simulink model "Micro_PMU_model"  (R2020b)
settings: Solver=VariableStepAuto  StartTime=0.0  StopTime=2  RelTol=1e-3  EnableMultiTasking=on
undefined symbols (not defined in the file): j, magnitude
libraries: powerlib_meascontrol x15, dsparch4 x3, dspsigops x3, powerlib x1
(part 1 of 3)
settings Model: Creator=Ahmed A.Elaziz  LastModifiedBy=Electronica Care
settings DataIOCC: ReturnWorkspaceOutputs=off
settings OptimizationCC: LifeSpan=inf
settings DebuggingCC: SFUnexpectedBacktrackingDiag=warning  SFNoUnconditionalDefaultTransitionDiag=warning  ArithmeticOperatorsInVariantConditions=warning
settings SFSimCC: SimUseLocalCustomCode=off  CustomCodeUndefinedFunction=UseInterfaceOnly
settings RTWCC: RTWUseLocalCustomCode=off
settings CodeAppCC: StateflowObjectComments=on
settings GRTTargetCC: TargetLangStandard=C89/C90 (ANSI)
settings ConfigComp: CovMetricSettings=dw  CovSaveCumulativeToWorkspaceVar=on  CovSaveSingleToWorkspaceVar=on  CovExternalEMLEnable=off

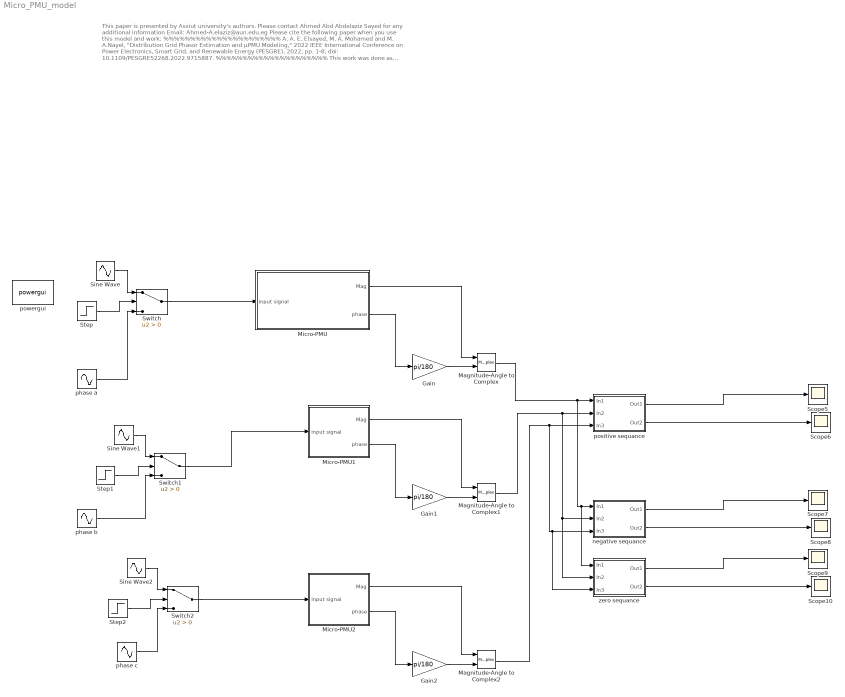
== system Micro_PMU_model ==
  note: This paper is presented by Assiut university's authors.
      | Please contact Ahmed Abd Abdelaziz Sayed for any additional information
      | Email: Ahmed-A.elaziz@aun.edu.eg
      |
      | Please cite the following paper when you use this model and work:
      | %%%%%%%%%%%%%%%%%%%%%%
      | A. A. E. Elsayed, M. A. Mohamed and M. A.Nayel,
      | "Distribution Grid Phasor Estimation and μPMU Modeling,"
      | 2022 IEEE International Conference on Power Electronics, Smart Grid, and Renewable Energy (PESGRE),
      | 2022, pp. 1-8, doi: 10.1109/PESGRE52268.2022.9715887.
      | %%%%%%%%%%%%%%%%%%%%%
      | This work was done as part of the research project “
      | Smart Monitoring system for Distribution Power Grid ”
      | supported by the Egyptian National Telecom Regulatory
      | Authority (NTRA).
      |
      | I hope this model and material are useful for you!!
      | Best wishes.
  Gain : Gain  Gain=pi/180
  Gain1 : Gain  Gain=pi/180
  Gain2 : Gain  Gain=pi/180
  Magnitude-Angle to Complex : MagnitudeAngleToComplex
  Magnitude-Angle to Complex1 : MagnitudeAngleToComplex
  Magnitude-Angle to Complex2 : MagnitudeAngleToComplex
  Micro-PMU : Subsystem
      mask Display: image('C:\Users\Ahmed A.Elaziz\Desktop\microPMU.png');
  Micro-PMU1 : Subsystem
      mask Display: image('C:\Users\Ahmed A.Elaziz\Desktop\microPMU.png');
  Micro-PMU2 : Subsystem
      mask Display: image('C:\Users\Ahmed A.Elaziz\Desktop\microPMU.png');
  Scope{5..10} (6 alike) : Scope
  Sine Wave : Sin  Frequency=2*pi*60  Phase=0/180*pi  SampleTime=0
  Sine Wave1 : Sin  Frequency=2*pi*60  Phase=-120/180*pi  SampleTime=0
  Sine Wave2 : Sin  Frequency=2*pi*60  Phase=120/180*pi  SampleTime=0
  Step : Step  Before=1  After=0  SampleTime=0
  Step1 : Step  Before=1  After=0  SampleTime=0
  Step2 : Step  Before=1  After=0  SampleTime=0
  Switch : Switch  Criteria=u2 > Threshold
  Switch1 : Switch  Criteria=u2 > Threshold
  Switch2 : Switch  Criteria=u2 > Threshold
  negative sequance : Subsystem
  phase a : Sin  Frequency=2*pi*59  Phase=0/180*pi  SampleTime=0
  phase b : Sin  Frequency=2*pi*59  Phase=-120/180*pi  SampleTime=0
  phase c : Sin  Frequency=2*pi*59  Phase=120/180*pi  SampleTime=0
  "positive sequance " : Subsystem
  powergui : powerlib/powergui  Priority=1  SimulationMode=Continuous  SampleTime=50e-6  frequency=60  Iterations=50  frequencyindice=60  Pbase=100e6  ErrMax=1e-4  UnitsV=kV  UnitsW=MW  buscounter=0  FunctionMessages=off  echomessages=off  EnableUseOfTLC=off  CurrentSourceSwitches=off  DisableSnubberDevices=off  DisableRonSwitches=off  DisableVfSwitches=off  DisplayEquations=off  AutomaticDiscreteSolvers=off  SolverType=Tustin/Backward Euler (TBE)  Interpol=off  ExternalGateDelay=off  methode=off  Ts=10  x0status=blocks  SPID=off  SwTol=0  HookPort=off  NonlinearTolerance=1e-4  nMaxIteration=100  ContinueOnMaxIteration=off  RestoreLinks=warning  ResistiveCurrentMeasurement=off  Frange=[0:2:500]  Ylog=off  Xlog=on  ShowGrid=off  save=off  variable=ZData  structure=0  ZoomFFT=off  StartTime=0.0  cycles=1  DisplayStyle=1  fundamental=60  FreqAxis=off  MaxFrequency=1000  frequencyindicesteady=1  RmsSteady=1  display=off
  "zero sequance " : Subsystem
  wires:
  Sine Wave1/1 -> Switch1/1
  "positive sequance "/1(Out1) -> Scope5/1
  Micro-PMU1/2(phase) -> Gain1/1
  Step/1 -> Switch/2
  Micro-PMU1/1(Mag) -> Magnitude-Angle to Complex1/1
  Micro-PMU/2(phase) -> Gain/1
  Sine Wave/1 -> Switch/1
  Gain2/1 -> Magnitude-Angle to Complex2/2
  Micro-PMU/1(Mag) -> Magnitude-Angle to Complex/1
  Gain1/1 -> Magnitude-Angle to Complex1/2
  negative sequance/1(Out1) -> Scope7/1
  Magnitude-Angle to Complex1/1 -> "zero sequance "/2(In2), negative sequance/2(In2), "positive sequance "/2(In2)
  Magnitude-Angle to Complex2/1 -> "zero sequance "/3(In3), negative sequance/3(In3), "positive sequance "/3(In3)
  "positive sequance "/2(Out2) -> Scope6/1
  Magnitude-Angle to Complex/1 -> "zero sequance "/1(In1), negative sequance/1(In1), "positive sequance "/1(In1)
  "zero sequance "/1(Out1) -> Scope9/1
  Step2/1 -> Switch2/2
  "zero sequance "/2(Out2) -> Scope10/1
  negative sequance/2(Out2) -> Scope8/1
  phase c/1 -> Switch2/3
  Step1/1 -> Switch1/2
  Switch2/1 -> Micro-PMU2/1(input signal)
  Sine Wave2/1 -> Switch2/1
  phase a/1 -> Switch/3
  Switch1/1 -> Micro-PMU1/1(input signal)
  Micro-PMU2/2(phase) -> Gain2/1
  Switch/1 -> Micro-PMU/1(input signal)
  phase b/1 -> Switch1/3
  Gain/1 -> Magnitude-Angle to Complex/2
  Micro-PMU2/1(Mag) -> Magnitude-Angle to Complex2/1

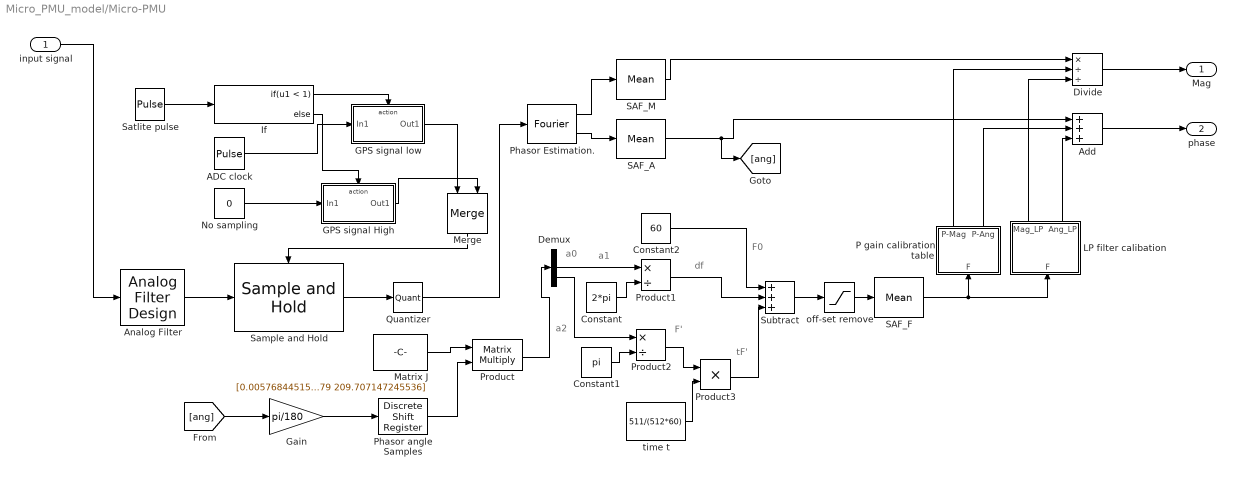
== system Micro_PMU_model/Micro-PMU ==
  note: F'
  note: a2
  note: F0
  note: tF'
  note: df
  note: a1
  note: a0
  input signal : Inport
  ADC clock : DiscretePulseGenerator  PulseType=Time based  Period=1/(60*512)
  Add : Sum  Inputs=+++
  Analog Filter : dsparch4/Analog Filter Design  method=Butterworth  filttype=Lowpass  N=2  Wlo=0.45*(2*pi*512*60)  Whi=80*2*pi  Rp=2  Rs=40
  Constant : Constant  Value=2*pi
  Constant1 : Constant  Value=pi
  Constant2 : Constant  Value=60
  Demux : Demux  Outputs=3
  Divide : Product  Inputs=*//
  GPS signal High : Subsystem  TreatAsAtomicUnit=on
  GPS signal low : Subsystem  TreatAsAtomicUnit=on
  Gain : Gain  Gain=pi/180
  If : If  IfExpression=u1 < 1
  LP filter calibation : Subsystem
  Matrix J : Constant  Value=|
      | [0.00576844515837218	0.00567795974412320	0.00558791875725266	0.00549832219776055	0.00540917006564686	0.00532046236091163	0.00523219908355482	0.00514438023357644	0.00505700581097649	0.00497007581575498	0.00488359024791190	0.00479754910744726	0.00471195239436104	0.00462680010865327	0.00454209225032392	0.00445782881937300	0.00437400981580053	0.00429063523960647	0.00420770509079087	0.00412521936935368	0.00404317807529494	0.00396158120861461	0.00388042876931273	0.00379972075738929	0.00371945717284428	0.00363963801567770	0.00356026328588955	0.00348133298347983	0.00340284710844855	0.00332480566079569	0.00324720864052127	0.00317005604762530	0.00309334788210774	0.00301708414396863	0.00294126483320794	0.00286588994982569	0.00279095949382187	0.00271647346519648	0.00264243186394953	0.00256883469008101	0.00249568194359093	0.00242297362447928	0.00235070973274606	0.00227889026839127	0.00220751523141491	0.00213658462181699	0.00206609843959751	0.00199605668475645	0.00192645935729383	0.00185730645720965	0.00178859798450389	0.00172033393917657	0.00165251432122768	0.00158513913065722	0.00151820836746520	0.00145172203165161	0.00138568012321645	0.00132008264215973	0.00125492958848144	0.00119022096218158	0.00112595676326016	0.00106213699171717	0.000998761647552607	0.000935830730766486	0.000873344241358794	0.000811302179329531	0.000749704544678715	0.000688551337406316	0.000627842557512357	0.000567578204996832	0.000507758279859736	0.000448382782101075	0.000389451711720848	0.000330965068719055	0.000272922853095699	0.000215325064850770	0.000158171703984276	0.000101462770496216	4.51982643865856e-05	-1.06218143446105e-05	-6.59974656973721e-05	-0.000120928689671705	-0.000175415486267602	-0.000229457855485058	-0.000283055797324093	-0.000336209311784687	-0.000388918398866853	-0.000441183058570583	-0.000493003290895880	-0.000544379095842747	-0.000595310473411180	-0.000645797423601178	-0.000695839946412735	-0.000745438041845870	-0.000794591709900570	-0.000843300950576835	-0.000891565763874672	-0.000939386149794073	-0.000986762108335040	-0.00103369363949757	-0.00108018074328167	-0.00112622341968733	-0.00117182166871457	-0.00121697549036337	-0.00126168488463374	-0.00130594985152568	-0.00134977039103918	-0.00139314650317425	-0.00143607818793089	-0.00147856544530908	-0.00152060827530885	-0.00156220667793019	-0.00160336065317310	-0.00164407020103756	-0.00168433532152361	-0.00172415601463121	-0.00176353228036038	-0.00180246411871111	-0.00184095152968342	-0.00187899451327729	-0.00191659306949273	-0.00195374719832974	-0.00199045689978831	-0.00202672217386845	-0.00206254302057016	-0.00209791943989343	-0.00213285143183826	-0.00216733899640467	-0.00220138213359265	-0.00223498084340219	-0.00226813512583330	-0.00230084498088597	-0.00233311040856022	-0.00236493140885603	-0.00239630798177339	-0.00242724012731234	-0.00245772784547285	-0.00248777113625492	-0.00251736999965857	-0.00254652443568378	-0.00257523444433055	-0.00260350002559890	-0.00263132117948881	-0.00265869790600028	-0.00268563020513333	-0.00271211807688794	-0.00273816152126412	-0.00276376053826187	-0.00278891512788118	-0.00281362529012206	-0.00283789102498450	-0.00286171233246851	-0.00288508921257409	-0.00290802166530124	-0.00293050969064995	-0.00295255328862023	-0.00297415245921208	-0.00299530720242550	-0.00301601751826048	-0.00303628340671703	-0.00305610486779514	-0.00307548190149483	-0.00309441450781607	-0.00311290268675889	-0.00313094643832327	-0.00314854576250922	-0.00316570065931674	-0.00318241112874582	-0.00319867717079647	-0.00321449878546869	-0.00322987597276247	-0.00324480873267782	-0.00325929706521474	-0.00327334097037323	-0.00328694044815328	-0.00330009549855489	-0.00331280612157808	-0.00332507231722283	-0.00333689408548915	-0.00334827142637704	-0.00335920433988649	-0.00336969282601751	-0.00337973688477010	-0.00338933651614426	-0.00339849172013997	-0.00340720249675726	-0.00341546884599612	-0.00342329076785654	-0.00343066826233853	-0.00343760132944208	-0.00344408996916721	-0.00345013418151389	-0.00345573396648215	-0.00346088932407197	-0.00346560025428336	-0.00346986675711632	-0.00347368883257084	-0.00347706648064693	-0.00347999970134459	-0.00348248849466382	-0.00348453286060461	-0.00348613279916697	-0.00348728831035089	-0.00348799939415638	-0.00348826605058344	-0.00348808827963207	-0.00348746608130226	-0.00348639945559402	-0.00348488840250735	-0.00348293292204224	-0.00348053301419870	-0.00347768867897673	-0.00347439991637632	-0.00347066672639749	-0.00346648910904021	-0.00346186706430451	-0.00345680059219037	-0.00345128969269780	-0.00344533436582679	-0.00343893461157735	-0.00343209042994949	-0.00342480182094318	-0.00341706878455844	-0.00340889132079527	-0.00340026942965367	-0.00339120311113364	-0.00338169236523517	-0.00337173719195827	-0.00336133759130293	-0.00335049356326916	-0.00333920510785696	-0.00332747222506632	-0.00331529491489726	-0.00330267317734976	-0.00328960701242383	-0.00327609642011946	-0.00326214140043666	-0.00324774195337542	-0.00323289807893576	-0.00321760977711766	-0.00320187704792113	-0.00318569989134616	-0.00316907830739277	-0.00315201229606094	-0.00313450185735067	-0.00311654699126197	-0.00309814769779484	-0.00307930397694928	-0.00306001582872528	-0.00304028325312285	-0.00302010625014199	-0.00299948481978269	-0.00297841896204496	-0.00295690867692880	-0.00293495396443420	-0.00291255482456117	-0.00288971125730971	-0.00286642326267981	-0.00284269084067149	-0.00281851399128473	-0.00279389271451954	-0.00276882701037590	-0.00274331687885384	-0.00271736231995335	-0.00269096333367443	-0.00266411992001706	-0.00263683207898127	-0.00260909981056705	-0.00258092311477439	-0.00255230199160330	-0.00252323644105377	-0.00249372646312581	-0.00246377205781942	-0.00243337322513460	-0.00240252996507134	-0.00237124227762965	-0.00233951016280953	-0.00230733362061097	-0.00227471265103398	-0.00224164725407856	-0.00220813742974470	-0.00217418317803241	-0.00213978449894169	-0.00210494139247253	-0.00206965385862495	-0.00203392189739893	-0.00199774550879447	-0.00196112469281158	-0.00192405944945026	-0.00188654977871051	-0.00184859568059232	-0.00181019715509570	-0.00177135420222065	-0.00173206682196716	-0.00169233501433524	-0.00165215877932489	-0.00161153811693611	-0.00157047302716889	-0.00152896351002324	-0.00148700956549915	-0.00144461119359663	-0.00140176839431568	-0.00135848116765630	-0.00131474951361848	-0.00127057343220223	-0.00122595292340755	-0.00118088798723443	-0.00113537862368288	-0.00108942483275290	-0.00104302661444449	-0.000996183968757638	-0.000948896895692355	-0.000901165395248640	-0.000852989467426492	-0.000804369112225912	-0.000755304329646896	-0.000705795119689450	-0.000655841482353571	-0.000605443417639258	-0.000554600925546511	-0.000503314006075330	-0.000451582659225718	-0.000399406884997672	-0.000346786683391194	-0.000293722054406281	-0.000240212998042937	-0.000186259514301160	-0.000131861603180946	-7.70192646823030e-05	-2.17324988052252e-05	3.39986944502843e-05	9.01743150842284e-05	0.000146794363096604	0.000203858838487415	0.000261367741256657	0.000319321071404334	0.000377718828930443	0.000436561013834986	0.000495847626117961	0.000555578665779368	0.000615754132819209	0.000676374027237483	0.000737438349034192	0.000798947098209333	0.000860900274762906	0.000923297878694913	0.000986139910005353	0.00104942636869423	0.00111315725476153	0.00117733256820727	0.00124195230903144	0.00130701647723405	0.00137252507281509	0.00143847809577456	0.00150487554611246	0.00157171742382880	0.00163900372892357	0.00170673446139678	0.00177490962124841	0.00184352920847848	0.00191259322308699	0.00198210166507392	0.00205205453443929	0.00212245183118309	0.00219329355530533	0.00226457970680600	0.00233631028568510	0.00240848529194264	0.00248110472557860	0.00255416858659300	0.00262767687498584	0.00270162959075711	0.00277602673390681	0.00285086830443494	0.00292615430234151	0.00300188472762650	0.00307805958028994	0.00315467886033180	0.00323174256775210	0.00330925070255083	0.00338720326472800	0.00346560025428360	0.00354444167121763	0.00362372751553009	0.00370345778722099	0.00378363248629032	0.00386425161273808	0.00394531516656428	0.00402682314776891	0.00410877555635197	0.00419117239231347	0.00427401365565340	0.00435729934637176	0.00444102946446856	0.00452520400994378	0.00460982298279744	0.00469488638302954	0.00478039421064007	0.00486634646562903	0.00495274314799642	0.00503958425774225	0.00512686979486651	0.00521459975936920	0.00530277415125033	0.00539139297050989	0.00548045621714788	0.00556996389116430	0.00565991599255916	0.00575031252133246	0.00584115347748418	0.00593243886101434	0.00602416867192293	0.00611634291020995	0.00620896157587541	0.00630202466891930	0.00639553218934162	0.00648948413714238	0.00658388051232157	0.00667872131487919	0.00677400654481525	0.00686973620212973	0.00696591028682266	0.00706252879889401	0.00715959173834380	0.00725709910517202	0.00735505089937867	0.00745344712096376	0.00755228776992728	0.00765157284626924	0.00775130234998962	0.00785147628108844	0.00795209463956569	0.00805315742542138	0.00815466463865550	0.00825661627926805	0.00835901234725904	0.00846185284262845	0.00856513776537630	0.00866886711550259	0.00877304089300731	0.00887765909789046	0.00898272173015204	0.00908822878979206	0.00919418027681051	0.00930057619120739	0.00940741653298270	0.00951470130213646	0.00962243049866864	0.00973060412257925	0.00983922217386830	0.00994828465253578	0.0100577915585817	0.0101677428920060	0.0102781386528088	0.0103889788409900	0.0105002634565497	0.0106119924994878	0.0107241659698043	0.0108367838674992	0.0109498461925726	0.0110633529450244	0.0111773041248547	0.0112916997320633	0.0114065397666505	0.0115218242286160	0.0116375531179600	0.0117537264346824	0.0118703441787832	0.0119874063502625	0.0121049129491202	0.0122228639753564	0.0123412594289709	0.0124600993099639	0.0125793836183354	0.0126991123540853	0.0128192855172136	0.0129399031077203	0.0130609651256055	0.0131824715708691	0.0133044224435111	0.0134268177435316	0.0135496574709305	0.0136729416257079	0.0137966702078636	0.0139208432173978	0.0140454606543105	0.0141705225186016	0.0142960288102711	0.0144219795293190	0.0145483746757454	0.0146752142495502	0.0148024982507334	0.0149302266792951	0.0150583995352352	0.0151870168185537	0.0153160785292507	0.0154455846673261	0.0155755352327799	0.0157059302256122	0.0158367696458229	0.0159680534934120	0.0160997817683796	0.0162319544707256	0.0163645716004500	0.0164976331575529	0.0166311391420342	0.0167650895538940	0.0168994843931321	0.0170343236597487	0.0171696073537438	0.0173053354751172	0.0174415080238691
      | -2.78653833026131	-2.74832649557359	-2.71027528216899	-2.67238469004751	-2.63465471920915	-2.59708536965392	-2.55967664138181	-2.52242853439282	-2.48534104868696	-2.44841418426422	-2.41164794112461	-2.37504231926811	-2.33859731869474	-2.30231293940449	-2.26618918139737	-2.23022604467337	-2.19442352923249	-2.15878163507473	-2.12330036220010	-2.08797971060859	-2.05281968030021	-2.01782027127494	-1.98298148353280	-1.94830331707379	-1.91378577189790	-1.87942884800513	-1.84523254539548	-1.81119686406895	-1.77732180402555	-1.74360736526527	-1.71005354778812	-1.67666035159409	-1.64342777668318	-1.61035582305539	-1.57744449071073	-1.54469377964919	-1.51210368987078	-1.47967422137548	-1.44740537416331	-1.41529714823427	-1.38334954358834	-1.35156256022554	-1.31993619814587	-1.28847045734931	-1.25716533783588	-1.22602083960557	-1.19503696265839	-1.16421370699432	-1.13355107261339	-1.10304905951557	-1.07270766770088	-1.04252689716931	-1.01250674792086	-0.982647219955539	-0.952948313273338	-0.923410027874263	-0.894032363758310	-0.864815320925476	-0.835758899375770	-0.806863099109185	-0.778127920125725	-0.749553362425387	-0.721139426008170	-0.692886110874080	-0.664793417023112	-0.636861344455265	-0.609089893170544	-0.581479063168942	-0.554028854450466	-0.526739267015112	-0.499610300862882	-0.472641955993775	-0.445834232407792	-0.419187130104932	-0.392700649085192	-0.366374789348578	-0.340209550895087	-0.314204933724720	-0.288360937837475	-0.262677563233351	-0.237154809912353	-0.211792677874476	-0.186591167119723	-0.161550277648094	-0.136670009459586	-0.111950362554203	-0.0873913369319423	-0.0629929325928056	-0.0387551495367925	-0.0146779877639011	0.00923855272586846	0.0329944719325126	0.0565897698560331	0.0800244464964320	0.103298501853707	0.126411935927861	0.149364748718891	0.172156940226797	0.194788510451580	0.217259459393239	0.239569787051776	0.261719493427188	0.283708578519480	0.305537042328648	0.327204884854691	0.348712106097613	0.370058706057410	0.391244684734086	0.412270042127638	0.433134778238067	0.453838893065372	0.474382386609553	0.494765258870615	0.514987509848551	0.535049139543366	0.554950147955055	0.574690535083622	0.594270300929065	0.613689445491387	0.632947968770583	0.652045870766658	0.670983151479609	0.689759810909436	0.708375849056144	0.726831265919726	0.745126061500184	0.763260235797519	0.781233788811730	0.799046720542822	0.816699030990788	0.834190720155632	0.851521788037353	0.868692234635950	0.885702059951423	0.902551263983773	0.919239846733003	0.935767808199107	0.952135148382088	0.968341867281947	0.984387964898681	1.00027344123229	1.01599829628278	1.03156253005015	1.04696614253439	1.06220913373551	1.07729150365351	1.09221325228838	1.10697437964013	1.12157488570876	1.13601477049427	1.15029403399665	1.16441267621591	1.17837069715204	1.19216809680505	1.20580487517494	1.21928103226170	1.23259656806535	1.24575148258587	1.25874577582326	1.27157944777754	1.28425249844869	1.29676492783671	1.30911673594162	1.32130792276340	1.33333848830206	1.34520843255759	1.35691775553000	1.36846645721929	1.37985453762545	1.39108199674850	1.40214883458842	1.41305505114521	1.42380064641888	1.43438562040943	1.44480997311686	1.45507370454116	1.46517681468234	1.47511930354040	1.48490117111533	1.49452241740714	1.50398304241583	1.51328304614140	1.52242242858384	1.53140118974316	1.54021932961935	1.54887684821243	1.55737374552237	1.56571002154920	1.57388567629290	1.58190070975348	1.58975512193094	1.59744891282527	1.60498208243648	1.61235463076457	1.61956655780953	1.62661786357138	1.63350854805009	1.64023861124569	1.64680805315816	1.65321687378751	1.65946507313373	1.66555265119684	1.67147960797682	1.67724594347367	1.68285165768740	1.68829675061801	1.69358122226550	1.69870507262986	1.70366830171111	1.70847090950922	1.71311289602422	1.71759426125609	1.72191500520484	1.72607512787046	1.73007462925296	1.73391350935234	1.73759176816860	1.74110940570173	1.74446642195174	1.74766281691863	1.75069859060239	1.75357374300303	1.75628827412055	1.75884218395494	1.76123547250621	1.76346813977436	1.76554018575938	1.76745161046129	1.76920241388006	1.77079259601572	1.77222215686825	1.77349109643766	1.77459941472395	1.77554711172711	1.77633418744715	1.77696064188406	1.77742647503786	1.77773168690853	1.77787627749608	1.77786024680050	1.77768359482180	1.77734632155998	1.77684842701503	1.77618991118697	1.77537077407577	1.77439101568146	1.77325063600402	1.77194963504346	1.77048801279978	1.76886576927297	1.76708290446304	1.76513941836999	1.76303531099381	1.76077058233451	1.75834523239209	1.75575926116654	1.75301266865787	1.75010545486608	1.74703761979116	1.74380916343313	1.74042008579197	1.73687038686768	1.73316006666027	1.72928912516974	1.72525756239609	1.72106537833931	1.71671257299941	1.71219914637639	1.70752509847024	1.70269042928097	1.69769513880858	1.69253922705307	1.68722269401443	1.68174553969267	1.67610776408778	1.67030936719977	1.66435034902864	1.65823070957439	1.65195044883701	1.64550956681651	1.63890806351289	1.63214593892614	1.62522319305627	1.61813982590328	1.61089583746716	1.60349122774792	1.59592599674556	1.58820014446007	1.58031367089147	1.57226657603973	1.56405885990488	1.55569052248690	1.54716156378580	1.53847198380158	1.52962178253423	1.52061095998376	1.51143951615017	1.50210745103345	1.49261476463361	1.48296145695065	1.47314752798456	1.46317297773535	1.45303780620302	1.44274201338757	1.43228559928899	1.42166856390728	1.41089090724246	1.39995262929451	1.38885373006344	1.37759420954925	1.36617406775193	1.35459330467149	1.34285192030793	1.33094991466124	1.31888728773143	1.30666403951850	1.29428017002244	1.28173567924327	1.26903056718096	1.25616483383554	1.24313847920699	1.22995150329532	1.21660390610052	1.20309568762261	1.18942684786157	1.17559738681740	1.16160730449012	1.14745660087971	1.13314527598617	1.11867332980952	1.10404076234974	1.08924757360684	1.07429376358081	1.05917933227166	1.04390427967939	1.02846860580400	1.01287231064548	0.997115394203836	0.981197856479072	0.965119697471185	0.948880917180175	0.932481515606042	0.915921492748785	0.899200848608405	0.882319583184902	0.865277696478277	0.848075188488528	0.830712059215656	0.813188308659660	0.795503936820542	0.777658943698300	0.759653329292935	0.741487093604448	0.723160236632837	0.704672758378103	0.686024658840246	0.667215938019266	0.648246595915162	0.629116632527936	0.609826047857587	0.590374841904114	0.570763014667518	0.550990566147799	0.531057496344958	0.510963805258993	0.490709492889904	0.470294559237693	0.449719004302359	0.428982828083901	0.408086030582320	0.387028611797617	0.365810571729790	0.344431910378840	0.322892627744767	0.301192723827570	0.279332198627251	0.257311052143809	0.235129284377243	0.212786895327555	0.190283884994743	0.167620253378808	0.144796000479750	0.121811126297569	0.0986656308322644	0.0753595140838372	0.0518927760522871	0.0282654167376133	0.00447743613981635	-0.0194711657411037	-0.0435803889051463	-0.0678502333523123	-0.0922806990826013	-0.116871786096013	-0.141623494392549	-0.166535823972207	-0.191608774834989	-0.216842346980894	-0.242236540409922	-0.267791355122072	-0.293506791117346	-0.319382848395744	-0.345419526957264	-0.371616826801907	-0.397974747929674	-0.424493290340564	-0.451172454034576	-0.478012239011712	-0.505012645271971	-0.532173672815353	-0.559495321641858	-0.586977591751486	-0.614620483144238	-0.642423995820112	-0.670388129779110	-0.698512885021230	-0.726798261546474	-0.755244259354841	-0.783850878446331	-0.812618118820945	-0.841545980478681	-0.870634463419540	-0.899883567643523	-0.929293293150628	-0.958863639940857	-0.988594608014209	-1.01848619737068	-1.04853840801028	-1.07875123993300	-1.10912469313885	-1.13965876762782	-1.17035346339991	-1.20120878045512	-1.23222471879346	-1.26340127841492	-1.29473845931950	-1.32623626150721	-1.35789468497803	-1.38971372973199	-1.42169339576906	-1.45383368308926	-1.48613459169258	-1.51859612157903	-1.55121827274860	-1.58400104520129	-1.61694443893710	-1.65004845395604	-1.68331309025810	-1.71673834784328	-1.75032422671159	-1.78407072686302	-1.81797784829757	-1.85204559101525	-1.88627395501605	-1.92066294029997	-1.95521254686701	-1.98992277471718	-2.02479362385047	-2.05982509426689	-2.09501718596643	-2.13036989894909	-2.16588323321487	-2.20155718876378	-2.23739176559581	-2.27338696371096	-2.30954278310924	-2.34585922379064	-2.38233628575516	-2.41897396900280	-2.45577227353357	-2.49273119934747	-2.52985074644448	-2.56713091482462	-2.60457170448788	-2.64217311543426	-2.67993514766377	-2.71785780117640	-2.75594107597216	-2.79418497205103	-2.83258948941303	-2.87115462805816	-2.90988038798640	-2.94876676919777	-2.98781377169226	-3.02702139546988	-3.06638964053062	-3.10591850687448	-3.14560799450146	-3.18545810341157	-3.22546883360480	-3.26564018508116	-3.30597215784064	-3.34646475188324	-3.38711796720896	-3.42793180381781	-3.46890626170978	-3.51004134088487	-3.55133704134308	-3.59279336308442	-3.63441030610889	-3.67618787041647	-3.71812605600718	-3.76022486288101	-3.80248429103797	-3.84490434047804	-3.88748501120124	-3.93022630320757	-3.97312821649702	-4.01619075106959	-4.05941390692528	-4.10279768406410	-4.14634208248604	-4.19004710219110
      | 209.707147245538	207.244832405082	204.792173701255	202.349171134057	199.915824703488	197.492134409549	195.078100252238	192.673722231557	190.279000347506	187.893934600083	185.518524989290	183.152771515126	180.796674177591	178.450232976686	176.113447912409	173.786318984762	171.468846193744	169.161029539356	166.862869021597	164.574364640467	162.295516395966	160.026324288094	157.766788316852	155.516908482239	153.276684784255	151.046117222900	148.825205798175	146.613950510079	144.412351358612	142.220408343774	140.038121465566	137.865490723986	135.702516119037	133.549197650716	131.405535319024	129.271529123962	127.147179065529	125.032485143725	122.927447358551	120.832065710006	118.746340198090	116.670270822803	114.603857584145	112.547100482117	110.499999516718	108.462554687948	106.434765995808	104.416633440296	102.408157021414	100.409336739161	98.4201725935377	96.4406645845435	94.4708127121781	92.5106169764423	90.5600773773357	88.6191939148583	86.6879665890101	84.7663953997912	82.8544803472015	80.9522214312411	79.0596186519098	77.1766720092079	75.3033815031352	73.4397471336917	71.5857689008776	69.7414468046924	67.9067808451368	66.0817710222101	64.2664173359129	62.4607197862449	60.6646783732061	58.8782930967965	57.1015639570162	55.3344909538652	53.5770740873433	51.8293133574507	50.0912087641874	48.3627603075533	46.6439679875485	44.9348318041728	43.2353517574265	41.5455278473093	39.8653600738213	38.1948484369627	36.5339929367333	34.8827935731331	33.2412503461622	31.6093632558205	29.9871323021080	28.3745574850248	26.7716388045708	25.1783762607461	23.5947698535507	22.0208195829843	20.4565254490473	18.9018874517395	17.3569055910610	15.8215798670117	14.2959102795917	12.7798968288008	11.2735395146392	9.77683833710694	8.28979329620390	6.81240439193001	5.34467162428540	3.88659499327006	2.43817449888399	0.999410141127082	-0.429698080000565	-1.84915016449905	-3.25894611236815	-4.65908592360798	-6.04956959821890	-7.43039713620018	-8.80156853755244	-10.1630838022754	-11.5149429303691	-12.8571459218336	-14.1896927766688	-15.5125834948747	-16.8258180764516	-18.1293965213990	-19.4233188297172	-20.7075850014064	-21.9821950364662	-23.2471489348968	-24.5024466966980	-25.7480883218699	-26.9840738104129	-28.2104031623265	-29.4270763776108	-30.6340934562660	-31.8314543982918	-33.0191592036884	-34.1972078724558	-35.3656004045939	-36.5243368001029	-37.6734170589825	-38.8128411812329	-39.9426091668541	-41.0627210158460	-42.1731767282087	-43.2739763039422	-44.3651197430464	-45.4466070455213	-46.5184382113672	-47.5806132405836	-48.6331321331708	-49.6759948891288	-50.7092015084577	-51.7327519911572	-52.7466463372274	-53.7508845466684	-54.7454666194804	-55.7303925556628	-56.7056623552162	-57.6712760181402	-58.6272335444351	-59.5735349341007	-60.5101801871371	-61.4371693035442	-62.3545022833222	-63.2621791264707	-64.1601998329900	-65.0485644028803	-65.9272728361412	-66.7963251327728	-67.6557212927753	-68.5054613161484	-69.3455452028925	-70.1759729530072	-70.9967445664926	-71.8078600433489	-72.6093193835759	-73.4011225871736	-74.1832696541422	-74.9557605844814	-75.7185953781914	-76.4717740352722	-77.2152965557238	-77.9491629395461	-78.6733731867391	-79.3879272973029	-80.0928252712376	-80.7880671085429	-81.4736528092190	-82.1495823732658	-82.8158558006834	-83.4724730914718	-84.1194342456310	-84.7567392631609	-85.3843881440616	-86.0023808883330	-86.6107174959750	-87.2093979669881	-87.7984223013717	-88.3777904991263	-88.9475025602514	-89.5075584847473	-90.0579582726141	-90.5987019238516	-91.1297894384598	-91.6512208164389	-92.1629960577887	-92.6651151625091	-93.1575781306004	-93.6403849620625	-94.1135356568952	-94.5770302150989	-95.0308686366731	-95.4750509216183	-95.9095770699341	-96.3344470816207	-96.7496609566781	-97.1552186951062	-97.5511202969051	-97.9373657620747	-98.3139550906150	-98.6808882825262	-99.0381653378082	-99.3857862564608	-99.7237510384843	-100.052059683878	-100.370712192643	-100.679708564779	-100.979048800286	-101.268732899163	-101.548760861411	-101.819132687030	-102.079848376019	-102.330907928379	-102.572311344110	-102.804058623212	-103.026149765685	-103.238584771528	-103.441363640742	-103.634486373327	-103.817952969282	-103.991763428609	-104.155917751306	-104.310415937374	-104.455257986812	-104.590443899622	-104.715973675802	-104.831847315353	-104.938064818274	-105.034626184567	-105.121531414230	-105.198780507264	-105.266373463669	-105.324310283444	-105.372590966590	-105.411215513107	-105.440183922995	-105.459496196253	-105.469152332883	-105.469152332883	-105.459496196253	-105.440183922995	-105.411215513107	-105.372590966590	-105.324310283444	-105.266373463669	-105.198780507264	-105.121531414230	-105.034626184567	-104.938064818275	-104.831847315353	-104.715973675802	-104.590443899622	-104.455257986812	-104.310415937374	-104.155917751306	-103.991763428609	-103.817952969283	-103.634486373327	-103.441363640742	-103.238584771528	-103.026149765685	-102.804058623212	-102.572311344111	-102.330907928380	-102.079848376019	-101.819132687030	-101.548760861411	-101.268732899163	-100.979048800286	-100.679708564779	-100.370712192644	-100.052059683879	-99.7237510384846	-99.3857862564612	-99.0381653378085	-98.6808882825266	-98.3139550906155	-97.9373657620751	-97.5511202969054	-97.1552186951066	-96.7496609566785	-96.3344470816211	-95.9095770699345	-95.4750509216187	-95.0308686366737	-94.5770302150993	-94.1135356568958	-93.6403849620630	-93.1575781306009	-92.6651151625097	-92.1629960577891	-91.6512208164394	-91.1297894384604	-90.5987019238521	-90.0579582726146	-89.5075584847480	-88.9475025602520	-88.3777904991268	-87.7984223013723	-87.2093979669887	-86.6107174959758	-86.0023808883336	-85.3843881440622	-84.7567392631615	-84.1194342456316	-83.4724730914725	-82.8158558006841	-82.1495823732665	-81.4736528092197	-80.7880671085436	-80.0928252712382	-79.3879272973037	-78.6733731867399	-77.9491629395468	-77.2152965557245	-76.4717740352730	-75.7185953781922	-74.9557605844822	-74.1832696541429	-73.4011225871744	-72.6093193835767	-71.8078600433497	-70.9967445664935	-70.1759729530080	-69.3455452028933	-68.5054613161494	-67.6557212927762	-66.7963251327738	-65.9272728361421	-65.0485644028812	-64.1601998329910	-63.2621791264717	-62.3545022833230	-61.4371693035451	-60.5101801871380	-59.5735349341017	-58.6272335444361	-57.6712760181413	-56.7056623552172	-55.7303925556639	-54.7454666194813	-53.7508845466695	-52.7466463372285	-51.7327519911582	-50.7092015084587	-49.6759948891299	-48.6331321331719	-47.5806132405847	-46.5184382113682	-45.4466070455225	-44.3651197430475	-43.2739763039433	-42.1731767282098	-41.0627210158472	-39.9426091668552	-38.8128411812341	-37.6734170589837	-36.5243368001040	-35.3656004045951	-34.1972078724570	-33.0191592036896	-31.8314543982930	-30.6340934562671	-29.4270763776120	-28.2104031623277	-26.9840738104141	-25.7480883218713	-24.5024466966993	-23.2471489348980	-21.9821950364674	-20.7075850014076	-19.4233188297186	-18.1293965214004	-16.8258180764529	-15.5125834948761	-14.1896927766701	-12.8571459218349	-11.5149429303705	-10.1630838022768	-8.80156853755379	-7.43039713620161	-6.04956959822020	-4.65908592360951	-3.25894611236960	-1.84915016450046	-0.429698080002073	0.999410141125579	2.43817449888245	3.88659499326855	5.34467162428390	6.81240439192852	8.28979329620235	9.77683833710542	11.2735395146377	12.7798968287993	14.2959102795901	15.8215798670101	17.3569055910594	18.9018874517379	20.4565254490457	22.0208195829827	23.5947698535490	25.1783762607444	26.7716388045692	28.3745574850231	29.9871323021063	31.6093632558188	33.2412503461605	34.8827935731314	36.5339929367316	38.1948484369610	39.8653600738196	41.5455278473075	43.2353517574247	44.9348318041710	46.6439679875467	48.3627603075515	50.0912087641856	51.8293133574489	53.5770740873415	55.3344909538634	57.1015639570144	58.8782930967947	60.6646783732042	62.4607197862430	64.2664173359111	66.0817710222083	67.9067808451348	69.7414468046906	71.5857689008756	73.4397471336898	75.3033815031333	77.1766720092060	79.0596186519079	80.9522214312391	82.8544803471995	84.7663953997892	86.6879665890081	88.6191939148563	90.5600773773337	92.5106169764403	94.4708127121762	96.4406645845413	98.4201725935357	100.409336739159	102.408157021412	104.416633440294	106.434765995806	108.462554687946	110.499999516716	112.547100482115	114.603857584143	116.670270822801	118.746340198087	120.832065710003	122.927447358549	125.032485143723	127.147179065527	129.271529123960	131.405535319022	133.549197650714	135.702516119034	137.865490723984	140.038121465563	142.220408343772	144.412351358609	146.613950510076	148.825205798172	151.046117222898	153.276684784253	155.516908482236	157.766788316849	160.026324288092	162.295516395963	164.574364640464	166.862869021594	169.161029539354	171.468846193742	173.786318984760	176.113447912407	178.450232976683	180.796674177589	183.152771515123	185.518524989287	187.893934600081	190.279000347503	192.673722231555	195.078100252236	197.492134409546	199.915824703485	202.349171134054	204.792173701252	207.244832405079	209.707147245536]
  Merge : Merge
  No sampling : Constant  Value=0
  P gain calibration table : Subsystem
  "Phasor Estimation. " : powerlib_meascontrol/Measurements/Fourier  Freq=60  n=1  InInit=[0, 0]  Ts=1/(60*512)
  Phasor angle Samples : powerlib_meascontrol/Additional Components/Discrete Shift Register  NSamples=512  InitialValue=0  Ts=1/(512*60)
      settings: SourceProductBaseCode=PS
  Product : Product  Multiplication=Matrix(*)
  Product1 : Product  Inputs=*/
  Product2 : Product  Inputs=*/
  Product3 : Product  Inputs=**
  Quantizer : Quantizer  QuantizationInterval=1/(2^(16))
  SAF_A : powerlib_meascontrol/Measurements/Mean  Freq=2*60  Vinit=0  Ts=1/(512*60)
  SAF_F : powerlib_meascontrol/Measurements/Mean  Freq=2*60  Vinit=0  Ts=1/(512*60)
  SAF_M : powerlib_meascontrol/Measurements/Mean  Freq=2*60  Vinit=0  Ts=1/(512*60)
  Sample and Hold : dspsigops/Sample and Hold  trig=Rising edge  initCond=0  latchinput=off
  "Satlite pulse " : DiscretePulseGenerator  PulseType=Time based  Period=1  PulseWidth=abs(((1/6)*randn+(1/2))*1e-6)*100
  Subtract : Sum  Inputs=+++
  off-set remove : Saturate  UpperLimit=61  LowerLimit=59
  time t : Constant  Value=511/(512*60)
  Mag : Outport
  phase : Outport  Port=2
  wires:
  "Satlite pulse "/1 -> If/1
  Demux/3 -> Product2/1
  Divide/1 -> Mag/1
  Add/1 -> phase/1
  Product/1 -> Demux/1
  Constant/1 -> Product1/2
  Constant2/1 -> Subtract/1
  "Phasor Estimation. "/2 -> SAF_A/1
  time t/1 -> Product3/2
  Matrix J/1 -> Product/1
  Phasor angle Samples/1 -> Product/2
  Product2/1 -> Product3/1
  Constant1/1 -> Product2/2
  Product1/1 -> Subtract/2
  Quantizer/1 -> "Phasor Estimation. "/1
  Sample and Hold/1 -> Quantizer/1
  If/1 -> GPS signal low/Action
  ADC clock/1 -> GPS signal low/1(In1)
  If/2 -> GPS signal High/Action
  Analog Filter/1 -> Sample and Hold/1
  No sampling/1 -> GPS signal High/1(In1)
  GPS signal High/1(Out1) -> Merge/2
  GPS signal low/1(Out1) -> Merge/1
  Merge/1 -> Sample and Hold/Trigger
  Demux/2 -> Product1/1
  SAF_M/1 -> Divide/1
  [ang] -> Gain/1
  "Phasor Estimation. "/1 -> SAF_M/1
  Gain/1 -> Phasor angle Samples/1
  SAF_A/1 -> Add/1, [ang]
  Product3/1 -> Subtract/3
  Subtract/1 -> off-set remove/1
  input signal/1 -> Analog Filter/1
  SAF_F/1 -> LP filter calibation/1(F), P gain calibration table/1(F)
  off-set remove/1 -> SAF_F/1
  P gain calibration table/1(P-Mag) -> Divide/2
  LP filter calibation/1(Mag_LP) -> Divide/3
  P gain calibration table/2(P-Ang) -> Add/2
  LP filter calibation/2(Ang_LP) -> Add/3
